simulink model "edge_trigger4_falling"  (R2018a)
settings: Solver=FixedStepAuto  StartTime=0.0  StopTime=10.0  FixedStep=0.1  MaxStep=1  RelTol=1e-3
settings Model: Creator=86188  LastModifiedBy=86188

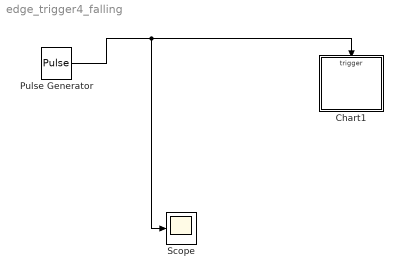
== system edge_trigger4_falling ==
  Chart1 : Stateflow chart  TreatAsAtomicUnit=on
  Pulse Generator : DiscretePulseGenerator  PulseType=Time based  Period=1  PulseWidth=50
  Scope : Scope
  wires:
  Pulse Generator/1 -> Scope/1, Chart1/Trigger

== stateflow chart edge_trigger4_falling/Chart1 ==
  state AA
    en:f("en_AA");
    du:f("du_AA");
  (default) -> AA : {y = y + 1;}
  data: s function_input; y local =0
  events: out_cmd input FALLING_EDGE_EVENT
  function f(s):
    | function f(s)
    |   fprintf(s+"\n");
